simulink model "quarterCarModel"  (R2026a)
settings: Solver=VariableStepAuto
values from neighbouring files (symbols this model uses):
  Cs = x(2)    [carConstraints.m]    (also in objectiveFunction.m; selectBestSolution.m = x(:,2))
  Ks = x(1)    [carConstraints.m]    (also in objectiveFunction.m; selectBestSolution.m = x(:,1))
  Kt = x(3)    [objectiveFunction.m]    (also in selectBestSolution.m = x(:,3))
  Ms = 70    [Parameter.m]    (also in carConstraints.m = evalin('base', 'Ms'); objectiveFunction.m = evalin('base', 'Ms'))
  Mu = 12.5    [Parameter.m]
settings Model: Creator=eonra  LastModifiedBy=eonra

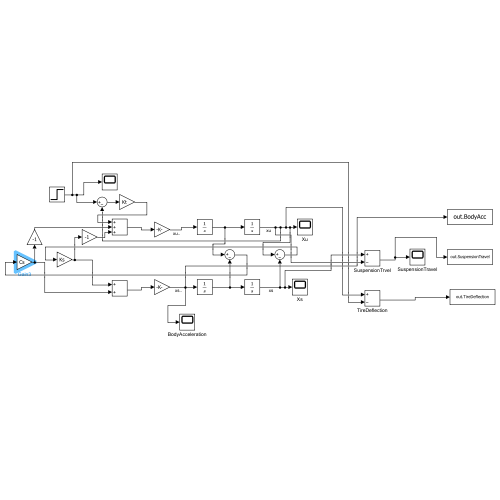
[thumbnail: Simulink's stored preview of the top-level diagram]
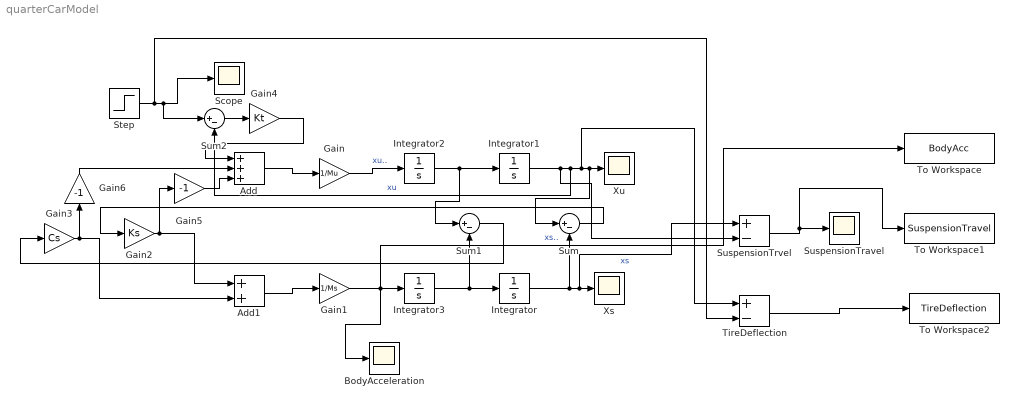
== system quarterCarModel ==
  Add : Sum  Inputs=+++
  Add1 : Sum
  BodyAcceleration : Scope
      settings: ActiveDisplayYMinimum=-61.171687061583754  ActiveDisplayYMaximum=122.00608839030943  DataLoggingVariableName=ScopeData3
  Gain : Gain  Gain=1/Mu
  Gain1 : Gain  Gain=1/Ms
  Gain2 : Gain  Gain=Ks
  Gain3 : Gain  Gain=Cs
  Gain4 : Gain  Gain=Kt
  Gain5 : Gain  Gain=-1
  Gain6 : Gain  Gain=-1
  Integrator{,1..3} (4 alike) : Integrator
  Scope : Scope
      settings: ActiveDisplayYMinimum=-1  ActiveDisplayYMaximum=1  DataLoggingVariableName=ScopeData2
  Step : Step  FinalValue=0.05  SampleTime=0
  Sum : Sum  Inputs=|+-
  Sum1 : Sum  Inputs=|+-
  Sum2 : Sum  Inputs=|+-
  SuspensionTravel : Scope
      settings: ActiveDisplayYMinimum=-0.030279916154888866  ActiveDisplayYMaximum=0.023424010409197872  DataLoggingVariableName=ScopeData4
  SuspensionTrvel : Sum  Inputs=+-
  TireDeflection : Sum  Inputs=+-
  To Workspace : ToWorkspace  VariableName=BodyAcc  SaveFormat=Timeseries  SampleTime=-1
  To Workspace1 : ToWorkspace  VariableName=SuspensionTravel  SaveFormat=Timeseries  SampleTime=-1
  To Workspace2 : ToWorkspace  VariableName=TireDeflection  SaveFormat=Timeseries  SampleTime=-1
  Xs : Scope
      settings: ActiveDisplayYMinimum=-0.083827848245272327  ActiveDisplayYMaximum=0.16196388793322791
  Xu : Scope
      settings: ActiveDisplayYMinimum=0.011776344736931621  ActiveDisplayYMaximum=0.0759611680155205
  wires:
  Integrator1/1 -> SuspensionTrvel/2, Sum2/2, TireDeflection/1, Sum/1, Xu/1  "xu"
  Integrator2/1 -> Sum1/1, Integrator1/1
  Integrator/1 -> SuspensionTrvel/1, Xs/1, Sum/2  "xs"
  Integrator3/1 -> Sum1/2, Integrator/1
  Gain/1 -> Integrator2/1  "xu.."
  Gain1/1 -> BodyAcceleration/1, To Workspace/1, Integrator3/1  "xs.."
  Sum/1 -> Gain2/1
  Gain2/1 -> Add1/1, Gain5/1
  Sum1/1 -> Gain3/1
  Gain3/1 -> Add1/2, Gain6/1
  Add1/1 -> Gain1/1
  Step/1 -> TireDeflection/2, Sum2/1, Scope/1
  Sum2/1 -> Gain4/1
  Gain4/1 -> Add/1
  Add/1 -> Gain/1
  Gain6/1 -> Add/2
  Gain5/1 -> Add/3
  SuspensionTrvel/1 -> To Workspace1/1, SuspensionTravel/1
  TireDeflection/1 -> To Workspace2/1
